simulink subsystem "PP_sub"  (R2024b)
settings: Solver=VariableStepAuto  StartTime=0.0  StopTime=10.0  RelTol=1e-3
undefined symbols (not defined in the file or in its folder): K1pp
libraries: cstblocks x1
settings Model: Creator=icpmoles  LastModifiedBy=icpmoles

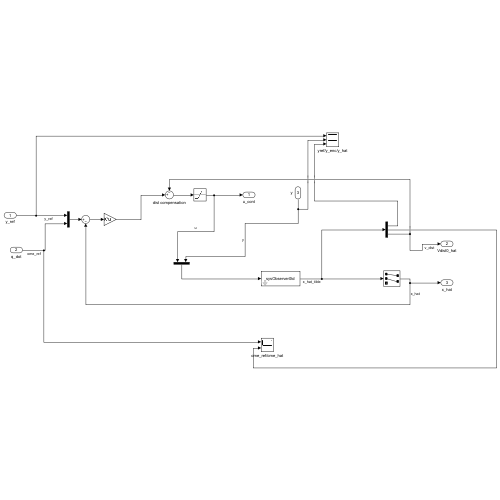
[thumbnail: Simulink's stored preview of the top-level diagram]
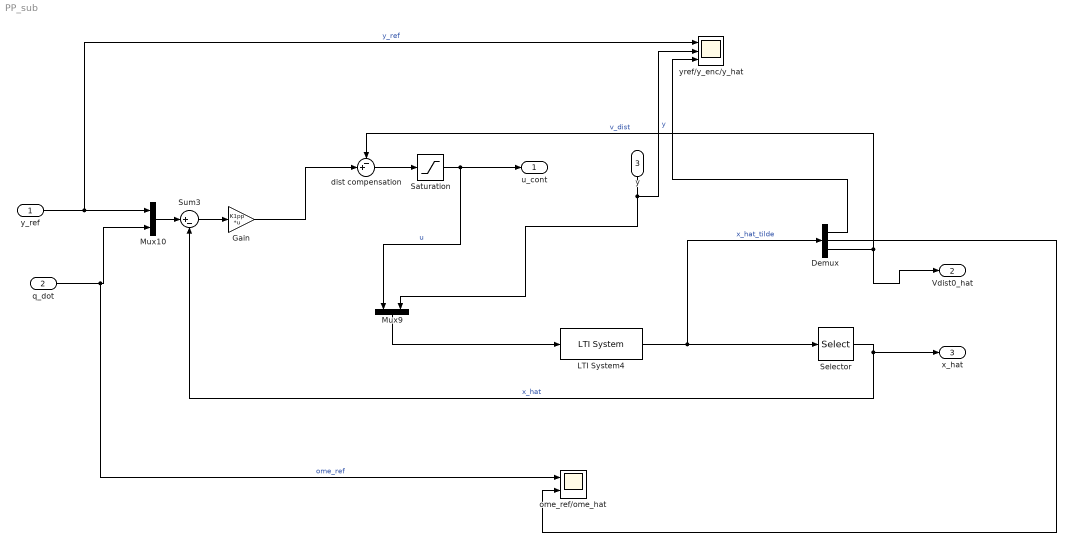
== system PP_sub ==
  y_ref : Inport
  q_dot : Inport  Port=2
  y : Inport  Port=3
  Demux : Demux  Outputs=3
  Gain : Gain  Gain=K1pp  Multiplication=Matrix(K*u)
  LTI System4 : cstblocks/LTI System  sys=sysObserver0td  IC=[]  PadeOrder=0
  Mux10 : Mux  Inputs=2
  Mux9 : Mux  Inputs=2
  Saturation : Saturate  UpperLimit=10  LowerLimit=-10
  Selector : Selector  InputPortWidth=3  IndexOptions=Index vector (dialog)  Indices=[1 2]  OutputSizes=1
  Sum3 : Sum  Inputs=|+-
  dist compensation : Sum  Inputs=-+|
  ome_ref/ome_hat : Scope  NumInputPorts=2
  yref/y_enc/y_hat : Scope  NumInputPorts=3
  u_cont : Outport
  Vdist0_hat : Outport  Port=2
  x_hat : Outport  Port=3
  wires:
  Mux9/1 -> LTI System4/1
  Saturation/1 -> u_cont/1, Mux9/1  "u"
  y/1 -> Mux9/2, yref/y_enc/y_hat/2  "y"
  Mux10/1 -> Sum3/1
  LTI System4/1 -> Demux/1, Selector/1  "x_hat_tilde"
  q_dot/1 -> ome_ref/ome_hat/1, Mux10/2  "ome_ref"
  Selector/1 -> x_hat/1, Sum3/2  "x_hat"
  dist compensation/1 -> Saturation/1
  Gain/1 -> dist compensation/2
  Demux/3 -> Vdist0_hat/1, dist compensation/1  "v_dist"
  Sum3/1 -> Gain/1
  y_ref/1 -> yref/y_enc/y_hat/1, Mux10/1  "y_ref"
  Demux/1 -> yref/y_enc/y_hat/3
  Demux/2 -> ome_ref/ome_hat/2
